simulink library "lib_env"  (Simulink 7.7)
settings: Solver=ode45  StartTime=0.0  StopTime=10.0  RelTol=1e-3
undefined symbols (not defined in the file): ADSW, area, arm, CD, CGP, CR, Earth, earth_radius, ele, GE, GGSW, GPperturbationSW, I, J2, jd, pSR, q_ini, rem_mag, rem_magSW, SGP, SRPSW, TOLERANCE, UT1_UTC, w_ini, wE, WGS84
libraries: lib_util x20, aerolibutil x13, lib_env x10, lib_orbittrance x9, aerolibtransform2 x6, lib_astrodynamics x5, aerolibatmos2 x1, vrlib x1, aerolibgravity2 x1
(part 1 of 2)
settings Model: Creator=kkamiya  LastModifiedBy=yamaurashusaku

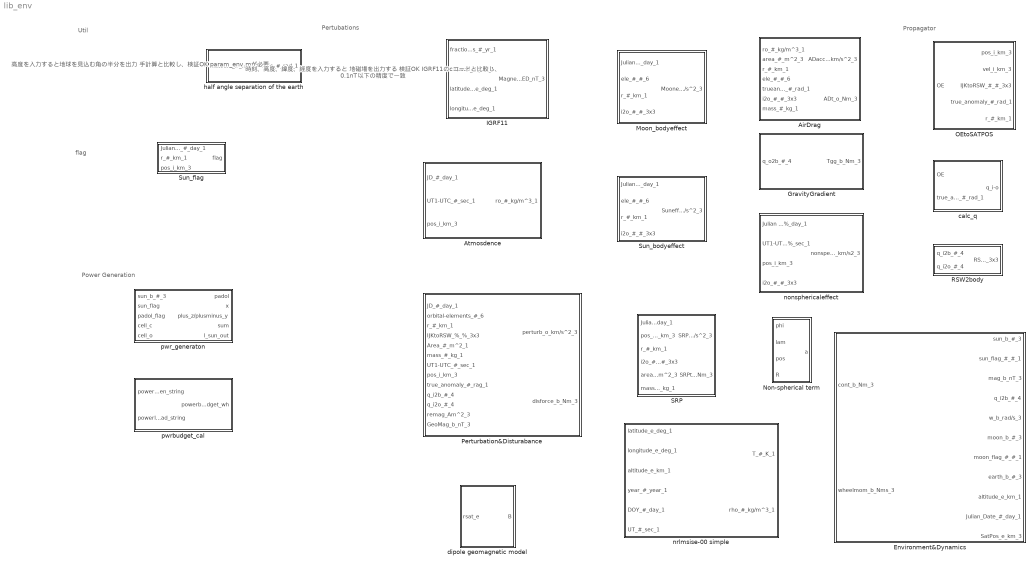
== system lib_env ==
  note: 高度を入力すると地球を見込む角の半分を出力
      | 手計算と比較し、検証OK
      | param_env.mが必要
  note: 時刻、高度、緯度、経度を入力すると
      | 地磁場を出力する
      | 検証OK
      | IGRF11のcコードと比較し、
      | 0.1nT以下の精度で一致
  note: Pertubations
  note: Util
  note: Propagator
  note: flag
  note: Power Generation
  AirDrag : Subsystem
  Atmosdence : Subsystem
  Environment&Dynamics : Subsystem
  GravityGradient : Subsystem
  IGRF11 : Subsystem
  Moon_bodyeffect : Subsystem
  Non-spherical term : Stateflow chart  TreatAsAtomicUnit=on
  OEtoSATPOS : Subsystem
  Perturbation&Disturabance : Subsystem
  RSW2body : Subsystem
  SRP : Subsystem
  Sun_bodyeffect : Subsystem
  Sun_flag : Subsystem
  calc_q : Subsystem
  dipole geomagnetic model : Stateflow chart  TreatAsAtomicUnit=on
  half angle separation of the earth : Subsystem
  nonsphericaleffect : Subsystem
  nrlmsise-00 simple : Subsystem
  pwr_generaton : Subsystem
  pwrbudget_cal : Subsystem

== system lib_env/AirDrag ==
  note: CD=2.2; arm=0.05cm
  ro_#_kg/m^3_1 : Inport
  area_#_m^2_3 : Inport  Port=2
  r_#_km_1 : Inport  Port=3
  ele_#_#_6 : Inport  Port=4
  trueanomaly_#_rad_1 : Inport  Port=5
  i2o_#_#_3x3 : Inport  Port=6
  mass_#_kg_1 : Inport  Port=7
  calc_AD : Stateflow chart  TreatAsAtomicUnit=on
  ADacc_o_km/s^2_3 : Outport
  ADt_o_Nm_3 : Outport  Port=2
  wires:
  calc_AD/1(AD_acc) -> ADacc_o_km/s^2_3/1
  calc_AD/2(AD_t) -> ADt_o_Nm_3/1
  ro_#_kg/m^3_1/1 -> calc_AD/1(ro)
  area_#_m^2_3/1 -> calc_AD/2(area)
  r_#_km_1/1 -> calc_AD/3(r)
  ele_#_#_6/1 -> calc_AD/4(ele)
  trueanomaly_#_rad_1/1 -> calc_AD/5(th)
  i2o_#_#_3x3/1 -> calc_AD/6(R)
  mass_#_kg_1/1 -> calc_AD/7(mass)

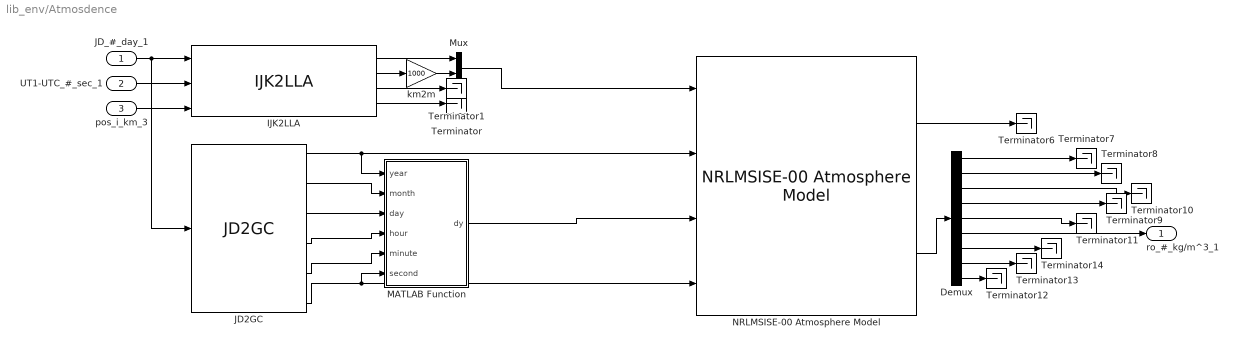
== system lib_env/Atmosdence ==
  JD_#_day_1 : Inport
  UT1-UTC_#_sec_1 : Inport  Port=2
  pos_i_km_3 : Inport  Port=3
  Demux : Demux  Outputs=9
  IJK2LLA : lib_orbittrance/IJK2LLA
  JD2GC : lib_util/JD2GC
  MATLAB Function : Stateflow chart  TreatAsAtomicUnit=on
  Mux : Mux  Inputs=2
  NRLMSISE-00 Atmosphere Model : aerolibatmos2/NRLMSISE-00 Atmosphere Model  units=Metric (MKS)  lst_input=off  flux_ap_input=off  flags_input=Internal  flags=ones(1,23)  oxygen_in=off  action=Warning
  Terminator{,1,6..14} (11 alike) : Terminator
  km2m : Gain  Gain=1000
  ro_#_kg/m^3_1 : Outport
  wires:
  IJK2LLA/1 -> Mux/1
  IJK2LLA/2 -> km2m/1
  km2m/1 -> Mux/2
  Mux/1 -> NRLMSISE-00 Atmosphere Model/1
  JD2GC/1 -> NRLMSISE-00 Atmosphere Model/2, MATLAB Function/1(year)
  JD2GC/6 -> NRLMSISE-00 Atmosphere Model/4, MATLAB Function/6(second)
  IJK2LLA/4 -> Terminator/1
  IJK2LLA/3 -> Terminator1/1
  JD2GC/2 -> MATLAB Function/2(month)
  JD2GC/3 -> MATLAB Function/3(day)
  JD2GC/4 -> MATLAB Function/4(hour)
  JD2GC/5 -> MATLAB Function/5(minute)
  JD_#_day_1/1 -> IJK2LLA/1, JD2GC/1
  UT1-UTC_#_sec_1/1 -> IJK2LLA/2
  pos_i_km_3/1 -> IJK2LLA/3
  NRLMSISE-00 Atmosphere Model/1 -> Terminator6/1
  NRLMSISE-00 Atmosphere Model/2 -> Demux/1
  Demux/6 -> ro_#_kg/m^3_1/1
  Demux/1 -> Terminator7/1
  Demux/2 -> Terminator8/1
  Demux/4 -> Terminator9/1
  Demux/3 -> Terminator10/1
  Demux/5 -> Terminator11/1
  Demux/9 -> Terminator12/1
  Demux/8 -> Terminator13/1
  Demux/7 -> Terminator14/1
  MATLAB Function/1(dy) -> NRLMSISE-00 Atmosphere Model/3

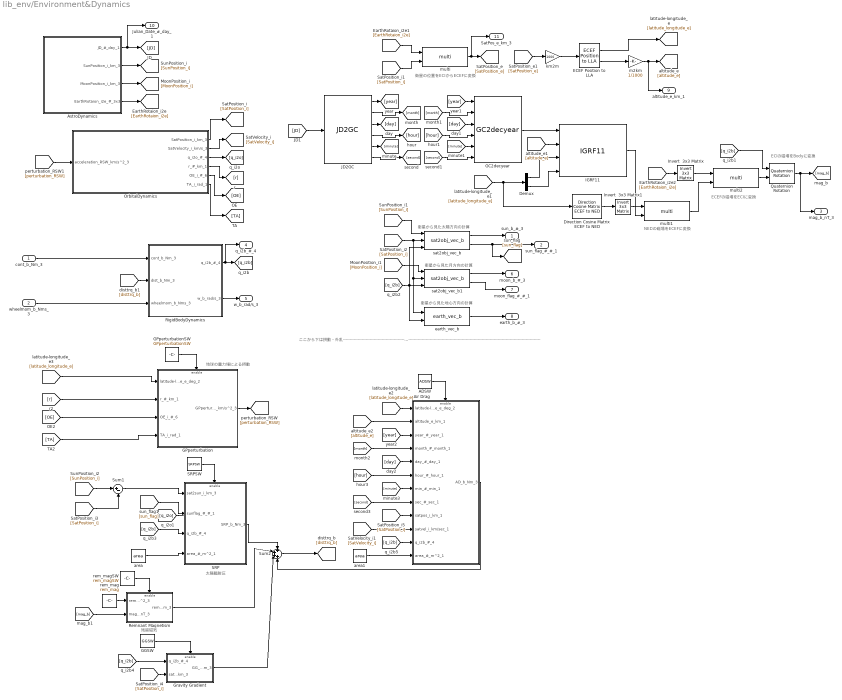
== system lib_env/Environment&Dynamics ==
  note: 残留磁気
  note: 太陽輻射圧
  note: 地球の重力場による摂動
  note: 衛星から見た地心方向の計算
  note: 衛星から見た月方向の計算
  note: 衛星から見た太陽方向の計算
  note: ECIの磁場をBodyに変換
  note: ECEFの磁場をECIに変換
  note: NEDの磁場をECEFに変換
  note: 衛星の位置をECIからECEFに変換
  note: ここから下は摂動・外乱-------------------------------------------------------------------------------------------------------------------------------------------------------------------------------------------------------------------------------------------------------------------------------------------------------------------------------------------------------
  cont_b_Nm_3 : Inport
  wheelmom_b_Nms_3 : Inport  Port=2
  ADSW : Constant  Value=ADSW
  Air Drag : Subsystem
  AstroDynamics : Subsystem
  Demux : Demux  Outputs=2
  Direction Cosine Matrix ECEF to NED : aerolibtransform2/Direction Cosine Matrix ECEF to NED  SystemSampleTime=-1
  ECEF Position to LLA : aerolibtransform2/ECEF Position to LLA  SystemSampleTime=-1  units=Metric (MKS)  ptype=Earth (WGS84)  F=1/298.257223563  R=6378137
  GC2decyear : lib_util/GC2decyear  SystemSampleTime=-1
  GGSW : Constant  Value=GGSW
  GPperturbation : Subsystem
  GPperturbationSW : Constant  Value=GPperturbationSW
  Gravity Gradient : Subsystem
  IGRF11 : lib_env/IGRF11  SystemSampleTime=-1
  Invert  3x3 Matrix : aerolibutil/Invert  3x3 Matrix  SystemSampleTime=-1
  Invert  3x3 Matrix1 : aerolibutil/Invert  3x3 Matrix  SystemSampleTime=-1
  JD2GC : lib_util/JD2GC  SystemSampleTime=-1
  OrbitalDynamics : Subsystem
  Quaternion Rotation : aerolibutil/Quaternion Rotation  SystemSampleTime=-1
  Remnant Magnetism : Subsystem
  RigidBodyDynamics : Subsystem
  SRP : Subsystem
  SRPSW : Constant  Value=SRPSW
  Sum1 : Sum  Inputs=|+-
  Sum2 : Sum  Inputs=++++
  area : Constant  Value=area
  area1 : Constant  Value=area
  earth_vec_b : lib_orbittrance/earth_vec_b  SystemSampleTime=-1
  km2m : Gain  Gain=1000
  m2km : Gain  Gain=1/1000
  multi : lib_util/multi  SystemSampleTime=-1
  multi1 : lib_util/multi  SystemSampleTime=-1
  multi2 : lib_util/multi  SystemSampleTime=-1
  rem_mag : Constant  Value=rem_mag
  rem_magSW : Constant  Value=rem_magSW
  sat2obj_vec_b : lib_orbittrance/sat2obj_vec_b  SystemSampleTime=-1
  sat2obj_vec_b1 : lib_orbittrance/sat2obj_vec_b  SystemSampleTime=-1
  sun_b_#_3 : Outport
  sun_flag_#_#_1 : Outport  Port=2
  mag_b_nT_3 : Outport  Port=3
  q_i2b_#_4 : Outport  Port=4
  w_b_rad/s_3 : Outport  Port=5
  moon_b_#_3 : Outport  Port=6
  moon_flag_#_#_1 : Outport  Port=7
  earth_b_#_3 : Outport  Port=8
  altitude_e_km_1 : Outport  Port=9
  Julian_Date_#_day_1 : Outport  Port=10
  SatPos_e_km_3 : Outport  Port=11
  wires:
  RigidBodyDynamics/2(w_b_rad/s_3) -> w_b_rad/s_3/1
  earth_vec_b/1 -> earth_b_#_3/1
  sat2obj_vec_b1/2 -> moon_flag_#_#_1/1
  sat2obj_vec_b1/1 -> moon_b_#_3/1
  sat2obj_vec_b/1 -> sun_b_#_3/1
  Air Drag/1(AD_b_Nm_3) -> Sum2/4
  ADSW/1 -> Air Drag/Enable
  [year] -> Air Drag/3(year_#_year_1)
  [q_i2b] -> Air Drag/11(q_i2b_#_4)
  area1/1 -> Air Drag/12(area_#_m^2_1)
  [SatVelocity_i] -> Air Drag/10(satvel_i_km/sec_1)
  [SatPosition_i] -> Air Drag/9(satpos_i_km_1)
  [second] -> Air Drag/8(sec_#_sec_1)
  [minute] -> Air Drag/7(min_#_min_1)
  [hour] -> Air Drag/6(hour_#_hour_1)
  [day] -> Air Drag/5(day_#_day_1)
  [month] -> Air Drag/4(month_#_month_1)
  [altitude_e] -> Air Drag/2(altitude_e_km_1)
  [latitude_longitude_e] -> Air Drag/1(latitude-longitude_e_deg_2)
  GGSW/1 -> Gravity Gradient/Enable
  [SatPosition_i] -> Gravity Gradient/2(satpos_i_km_3)
  [q_i2b] -> Gravity Gradient/1(q_i2b_#_4)
  SRP/1(SRP_b_Nm_3) -> Sum2/1
  [disttrq_b] -> RigidBodyDynamics/2(dist_b_Nm_3)
  Sum2/1 -> [disttrq_b]
  rem_magSW/1 -> Remnant Magnetism/Enable
  [mag_b] -> Remnant Magnetism/2(mag_b_nT_3)
  rem_mag/1 -> Remnant Magnetism/1(remmag_b_Am^2_3)
  SRPSW/1 -> SRP/Enable
  [SunPosition_i] -> Sum1/1
  [SatPosition_i] -> Sum1/2
  [q_i2b] -> SRP/3(q_i2b_#_4)
  [q_i2o] -> ?
  area/1 -> SRP/4(area_#_m^2_1)
  [sun_flag] -> SRP/2(sunflag_#_#_1)
  Sum1/1 -> SRP/1(sat2sun_i_km_3)
  sat2obj_vec_b/2 -> sun_flag_#_#_1/1, [sun_flag]
  [second] -> GC2decyear/6
  [minute] -> GC2decyear/5
  [hour] -> GC2decyear/4
  [day] -> GC2decyear/3
  [month] -> GC2decyear/2
  [year] -> GC2decyear/1
  JD2GC/6 -> [second]
  JD2GC/5 -> [minute]
  JD2GC/4 -> [hour]
  JD2GC/3 -> [day]
  JD2GC/2 -> [month]
  JD2GC/1 -> [year]
  GPperturbationSW/1 -> GPperturbation/Enable
  [TA] -> GPperturbation/4(TA_i_rad_1)
  [OE] -> GPperturbation/3(OE_i_#_6)
  [r] -> GPperturbation/2(r_#_km_1)
  [latitude_longitude_e] -> GPperturbation/1(latitude-longitude_e_deg_2)
  OrbitalDynamics/4(r_#_km_1) -> [r]
  OrbitalDynamics/6(TA_i_rad_1) -> [TA]
  OrbitalDynamics/5(OE_i_#_6) -> [OE]
  OrbitalDynamics/3(q_i2o_#_4) -> [q_i2o]
  [SunPosition_i] -> sat2obj_vec_b/1
  [MoonPosition_i] -> sat2obj_vec_b1/1
  [q_i2b] -> sat2obj_vec_b1/3, sat2obj_vec_b/3, earth_vec_b/2
  [SatPosition_i] -> sat2obj_vec_b/2, sat2obj_vec_b1/2, earth_vec_b/1
  Quaternion Rotation/1 -> mag_b_nT_3/1, [mag_b]
  [q_i2b] -> Quaternion Rotation/1
  RigidBodyDynamics/1(q_i2b_#_4) -> q_i2b_#_4/1, [q_i2b]
  multi2/1 -> Quaternion Rotation/2
  multi1/1 -> multi2/2
  Invert  3x3 Matrix/1 -> multi2/1
  [EarthRotaion_i2e] -> Invert  3x3 Matrix/1
  IGRF11/1 -> multi1/2
  Invert  3x3 Matrix1/1 -> multi1/1
  Direction Cosine Matrix ECEF to NED/1 -> Invert  3x3 Matrix1/1
  Demux/2 -> IGRF11/4
  Demux/1 -> IGRF11/3
  [altitude_e] -> IGRF11/2
  [latitude_longitude_e] -> Direction Cosine Matrix ECEF to NED/1, Demux/1
  [JD] -> JD2GC/1
  AstroDynamics/1(JD_#_day_1) -> Julian_Date_#_day_1/1, [JD]
  GC2decyear/1 -> IGRF11/1
  ECEF Position to LLA/1 -> [latitude_longitude_e]
  m2km/1 -> altitude_e_km_1/1, [altitude_e]
  ECEF Position to LLA/2 -> m2km/1
  km2m/1 -> ECEF Position to LLA/1
  [SatPosition_e] -> km2m/1
  multi/1 -> SatPos_e_km_3/1, [SatPosition_e]
  [SatPosition_i] -> multi/2
  [EarthRotaion_i2e] -> multi/1
  OrbitalDynamics/2(SatVelocity_i_km/s_3) -> [SatVelocity_i]
  OrbitalDynamics/1(SatPosition_i_km_3) -> [SatPosition_i]
  AstroDynamics/4(EarthRotaion_i2e_#_3x3) -> [EarthRotaion_i2e]
  AstroDynamics/3(MoonPosition_i_km_3) -> [MoonPosition_i]
  AstroDynamics/2(SunPosition_i_km_3) -> [SunPosition_i]
  wheelmom_b_Nms_3/1 -> RigidBodyDynamics/3(wheelmom_b_Nms_3)
  cont_b_Nm_3/1 -> RigidBodyDynamics/1(cont_b_Nm_3)
  Remnant Magnetism/1(remmag_b_Nm_3) -> Sum2/2
  Gravity Gradient/1(GG_b_Nm_3) -> Sum2/3
  GPperturbation/1(GPperturbation_RSW_km/s^2_3) -> [perturbation_RSW]
  [perturbation_RSW] -> OrbitalDynamics/1(acceleration_RSW_km/s^2_3)

== system lib_env/GravityGradient ==
  q_o2b_#_4 : Inport
  gravity_gradient : Stateflow chart  TreatAsAtomicUnit=on
  iInertiamatrix_#_kgm^2_3x3 : Constant  Value=I
  radius_vec : Stateflow chart  TreatAsAtomicUnit=on
  Tgg_b_Nm_3 : Outport
  wires:
  gravity_gradient/1(Tgg) -> Tgg_b_Nm_3/1
  radius_vec/1(ra_vec) -> gravity_gradient/1(ra)
  q_o2b_#_4/1 -> radius_vec/1(q)
  iInertiamatrix_#_kgm^2_3x3/1 -> gravity_gradient/2(I)

== system lib_env/IGRF11 ==
  fractional years_#_yr_1 : Inport
  altitude_#_km_1 : Inport  Port=2
  latitude_e_deg_1 : Inport  Port=3
  longitude_e_deg_1 : Inport  Port=4
  IGRF11 : Stateflow chart  TreatAsAtomicUnit=on
  Magnetic field_NED_nT_3 : Outport
  wires:
  fractional years_#_yr_1/1 -> IGRF11/1(fyears)
  altitude_#_km_1/1 -> IGRF11/2(alt)
  latitude_e_deg_1/1 -> IGRF11/3(nlat)
  longitude_e_deg_1/1 -> IGRF11/4(elong)
  IGRF11/1(B) -> Magnetic field_NED_nT_3/1

== system lib_env/Moon_bodyeffect ==
  JulianDate_#_day_1 : Inport
  ele_#_#_6 : Inport  Port=2
  r_#_km_1 : Inport  Port=3
  i2o_#_#_3x3 : Inport  Port=4
  moon position vector : lib_astrodynamics/moon position vector
  moonbodyeffect : Stateflow chart  TreatAsAtomicUnit=on
  Mooneff_o_km/s^2_3 : Outport
  wires:
  JulianDate_#_day_1/1 -> moon position vector/1
  r_#_km_1/1 -> moonbodyeffect/5(r)
  ele_#_#_6/1 -> moonbodyeffect/4(ele)
  i2o_#_#_3x3/1 -> moonbodyeffect/6(R)
  moonbodyeffect/1(F) -> Mooneff_o_km/s^2_3/1
  moon position vector/1 -> moonbodyeffect/1(lon)
  moon position vector/2 -> moonbodyeffect/2(lat)
  moon position vector/3 -> moonbodyeffect/3(rp)

== system lib_env/OEtoSATPOS ==
  OE : Inport
  calc_TA_R : Stateflow chart  TreatAsAtomicUnit=on
  sat_IJK : Stateflow chart  TreatAsAtomicUnit=on
  pos_i_km_3 : Outport
  vel_i_km_3 : Outport  Port=2
  IJKtoRSW_#_#_3x3 : Outport  Port=3
  true_anomaly_#_rad_1 : Outport  Port=4
  r_#_km_1 : Outport  Port=5
  wires:
  OE/1 -> calc_TA_R/1(OE)
  calc_TA_R/1(ele) -> sat_IJK/1(ele)
  calc_TA_R/2(th) -> sat_IJK/2(th), true_anomaly_#_rad_1/1
  calc_TA_R/3(r) -> sat_IJK/3(r), r_#_km_1/1
  calc_TA_R/4(R) -> sat_IJK/4(R), IJKtoRSW_#_#_3x3/1
  sat_IJK/1(pos) -> pos_i_km_3/1
  sat_IJK/2(v) -> vel_i_km_3/1

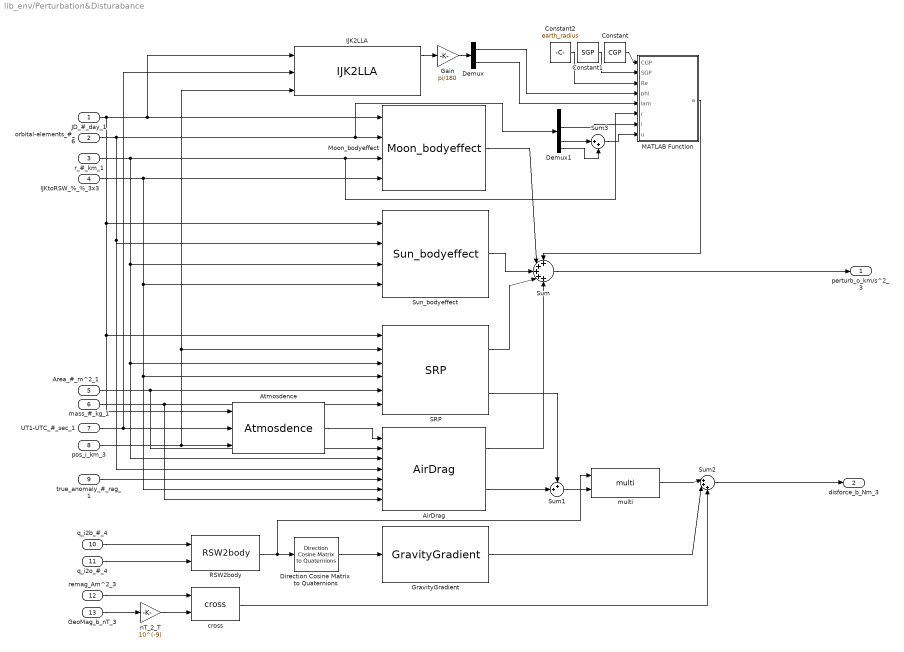
== system lib_env/Perturbation&Disturabance ==
  JD_#_day_1 : Inport
  orbital-elements_#_6 : Inport  Port=2
  r_#_km_1 : Inport  Port=3
  IJKtoRSW_%_%_3x3 : Inport  Port=4
  Area_#_m^2_1 : Inport  Port=5
  mass_#_kg_1 : Inport  Port=6
  UT1-UTC_#_sec_1 : Inport  Port=7
  pos_i_km_3 : Inport  Port=8
  true_anomaly_#_rag_1 : Inport  Port=9
  q_i2b_#_4 : Inport  Port=10
  q_i2o_#_4 : Inport  Port=11
  remag_Am^2_3 : Inport  Port=12
  GeoMag_b_nT_3 : Inport  Port=13
  AirDrag : lib_env/AirDrag
  Atmosdence : lib_env/Atmosdence
  Constant : Constant  Value=CGP
  Constant1 : Constant  Value=SGP
  Constant2 : Constant  Value=earth_radius
  Demux : Demux  Outputs=2
  Demux1 : Demux  Outputs=6
  Direction Cosine Matrix  to Quaternions : aerolibtransform2/Direction Cosine Matrix  to Quaternions
  Gain : Gain  Gain=pi/180
  GravityGradient : lib_env/GravityGradient
  IJK2LLA : lib_orbittrance/IJK2LLA
  MATLAB Function : Stateflow chart  TreatAsAtomicUnit=on
  Moon_bodyeffect : lib_env/Moon_bodyeffect
  RSW2body : lib_env/RSW2body
  SRP : lib_env/SRP
  Sum : Sum  Inputs=+++++
  Sum1 : Sum  Inputs=++|
  Sum2 : Sum  Inputs=|+++
  Sum3 : Sum  Inputs=|++
  Sun_bodyeffect : lib_env/Sun_bodyeffect
  cross : lib_util/cross
  multi : lib_util/multi
  nT_2_T : Gain  Gain=10^(-9)
  perturb_o_km/s^2_3 : Outport
  disforce_b_Nm_3 : Outport  Port=2
  wires:
  JD_#_day_1/1 -> Sun_bodyeffect/1, SRP/1, Atmosdence/1, Moon_bodyeffect/1, IJK2LLA/1
  orbital-elements_#_6/1 -> Sun_bodyeffect/2, AirDrag/4, Moon_bodyeffect/2, Demux1/1
  r_#_km_1/1 -> Sun_bodyeffect/3, SRP/3, AirDrag/3, Moon_bodyeffect/3, MATLAB Function/6(r)
  IJKtoRSW_%_%_3x3/1 -> Sun_bodyeffect/4, SRP/4, AirDrag/6, Moon_bodyeffect/4
  Area_#_m^2_1/1 -> SRP/5, AirDrag/2
  mass_#_kg_1/1 -> SRP/6, AirDrag/7
  true_anomaly_#_rag_1/1 -> AirDrag/5
  Sum/1 -> perturb_o_km/s^2_3/1
  SRP/2 -> Sum1/1
  AirDrag/2 -> Sum1/2
  Atmosdence/1 -> AirDrag/1
  UT1-UTC_#_sec_1/1 -> IJK2LLA/2, Atmosdence/2
  pos_i_km_3/1 -> Atmosdence/3, IJK2LLA/3, SRP/2
  q_i2b_#_4/1 -> RSW2body/1
  q_i2o_#_4/1 -> RSW2body/2
  RSW2body/1 -> Direction Cosine Matrix  to Quaternions/1, multi/1
  Direction Cosine Matrix  to Quaternions/1 -> GravityGradient/1
  GravityGradient/1 -> Sum2/2
  Sum1/1 -> multi/2
  multi/1 -> Sum2/1
  AirDrag/1 -> Sum/5
  SRP/1 -> Sum/4
  Sun_bodyeffect/1 -> Sum/3
  Moon_bodyeffect/1 -> Sum/2
  Sum2/1 -> disforce_b_Nm_3/1
  IJK2LLA/1 -> Gain/1
  Gain/1 -> Demux/1
  GeoMag_b_nT_3/1 -> nT_2_T/1
  nT_2_T/1 -> cross/2
  remag_Am^2_3/1 -> cross/1
  cross/1 -> Sum2/3
  Constant/1 -> MATLAB Function/1(CGP)
  Constant1/1 -> MATLAB Function/2(SGP)
  Constant2/1 -> MATLAB Function/3(Re)
  Demux/1 -> MATLAB Function/4(phi)
  Demux/2 -> MATLAB Function/5(lam)
  MATLAB Function/1(a) -> Sum/1
  Demux1/3 -> MATLAB Function/7(i)
  Demux1/5 -> Sum3/1
  Demux1/6 -> Sum3/2
  Sum3/1 -> MATLAB Function/8(u)

== system lib_env/RSW2body ==
  q_i2b_#_4 : Inport
  q_i2o_#_4 : Inport  Port=2
  Invert  3x3 Matrix : aerolibutil/Invert  3x3 Matrix
  Quaternions to  Direction Cosine Matrix : aerolibtransform2/Quaternions to  Direction Cosine Matrix
  Quaternions to  Direction Cosine Matrix1 : aerolibtransform2/Quaternions to  Direction Cosine Matrix
  multi : lib_util/multi
  RSW2b_#_#_3x3 : Outport
  wires:
  q_i2b_#_4/1 -> Quaternions to  Direction Cosine Matrix/1
  q_i2o_#_4/1 -> Quaternions to  Direction Cosine Matrix1/1
  Quaternions to  Direction Cosine Matrix1/1 -> Invert  3x3 Matrix/1
  Invert  3x3 Matrix/1 -> multi/2
  Quaternions to  Direction Cosine Matrix/1 -> multi/1
  multi/1 -> RSW2b_#_#_3x3/1

== system lib_env/SRP ==
  note: Arm=0.05cm
  JulianDate_#_day_1 : Inport
  pos_#_km_3 : Inport  Port=2
  r_#_km_1 : Inport  Port=3
  i2o_#_#_3x3 : Inport  Port=4
  area_#_m^2_3 : Inport  Port=5
  mass_#_kg_1 : Inport  Port=6
  srp : Stateflow chart  TreatAsAtomicUnit=on
  SRP_o_km/s^2_3 : Outport
  SRPt_o_Nm_3 : Outport  Port=2
  wires:
  r_#_km_1/1 -> srp/3(r)
  pos_#_km_3/1 -> srp/2(pos)
  i2o_#_#_3x3/1 -> srp/4(R)
  srp/1(SRP_acc) -> SRP_o_km/s^2_3/1
  JulianDate_#_day_1/1 -> srp/1(jd)
  area_#_m^2_3/1 -> srp/5(area)
  mass_#_kg_1/1 -> srp/6(mass)
  srp/2(SRP_t) -> SRPt_o_Nm_3/1

== system lib_env/Sun_bodyeffect ==
  JulianDate_#_day_1 : Inport
  ele_#_#_6 : Inport  Port=2
  r_#_km_1 : Inport  Port=3
  i2o_#_#_3x3 : Inport  Port=4
  Sun : lib_astrodynamics/sun position vector/Sun
  sun_b_e : Stateflow chart  TreatAsAtomicUnit=on
  Suneff_o_km/s^2_3 : Outport
  wires:
  Sun/1 -> sun_b_e/1(lon)
  Sun/2 -> sun_b_e/2(lat)
  Sun/3 -> sun_b_e/3(rp)
  r_#_km_1/1 -> sun_b_e/5(r)
  ele_#_#_6/1 -> sun_b_e/4(ele)
  i2o_#_#_3x3/1 -> sun_b_e/6(R)
  sun_b_e/1(F) -> Suneff_o_km/s^2_3/1
  JulianDate_#_day_1/1 -> Sun/1

== system lib_env/Sun_flag ==
  JulianDate_#_day_1 : Inport
  r_#_km_1 : Inport  Port=2
  pos_i_km_3 : Inport  Port=3
  srp : Stateflow chart  TreatAsAtomicUnit=on
  flag : Outport
  wires:
  pos_i_km_3/1 -> srp/2(pos)
  r_#_km_1/1 -> srp/3(r)
  srp/1(flag) -> flag/1
  JulianDate_#_day_1/1 -> srp/1(jd)

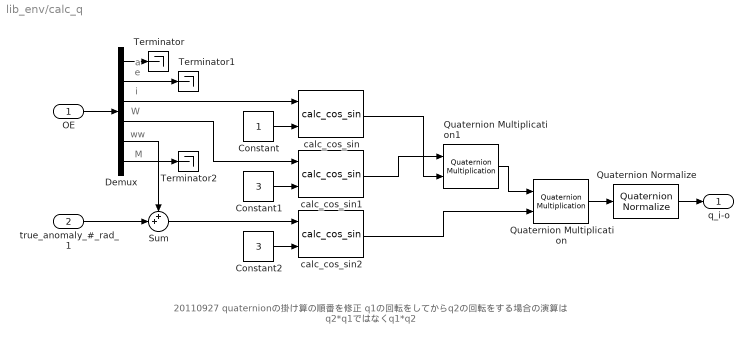
== system lib_env/calc_q ==
  note: M
  note: ww
  note: W
  note: i
  note: e
  note: a
  note: 20110927 quaternionの掛け算の順番を修正
      | q1の回転をしてからq2の回転をする場合の演算は
      | q2*q1ではなくq1*q2
  OE : Inport
  true_anomaly_#_rad_1 : Inport  Port=2
  Constant : Constant
  Constant1 : Constant  Value=3
  Constant2 : Constant  Value=3
  Demux : Demux  Outputs=6
  Quaternion Multiplication : aerolibutil/Quaternion Multiplication
  Quaternion Multiplication1 : aerolibutil/Quaternion Multiplication
  Quaternion Normalize : aerolibutil/Quaternion Normalize
  Sum : Sum  Inputs=++|
  Terminator : Terminator
  Terminator1 : Terminator
  Terminator2 : Terminator
  calc_cos_sin : lib_util/calc_cos_sin
  calc_cos_sin1 : lib_util/calc_cos_sin
  calc_cos_sin2 : lib_util/calc_cos_sin
  q_i-o : Outport
  wires:
  OE/1 -> Demux/1
  Quaternion Normalize/1 -> q_i-o/1
  true_anomaly_#_rad_1/1 -> Sum/2
  Demux/5 -> Sum/1
  Sum/1 -> calc_cos_sin2/1
  Demux/3 -> calc_cos_sin/1
  Demux/4 -> calc_cos_sin1/1
  Demux/1 -> Terminator/1
  Demux/2 -> Terminator1/1
  Demux/6 -> Terminator2/1
  Quaternion Multiplication/1 -> Quaternion Normalize/1
  Constant/1 -> calc_cos_sin/2
  Constant1/1 -> calc_cos_sin1/2
  Constant2/1 -> calc_cos_sin2/2
  calc_cos_sin1/1 -> Quaternion Multiplication1/1
  calc_cos_sin/1 -> Quaternion Multiplication1/2
  Quaternion Multiplication1/1 -> Quaternion Multiplication/1
  calc_cos_sin2/1 -> Quaternion Multiplication/2

== system lib_env/half angle separation of the earth ==
  altitude_#_km_1 : Inport
  MATLAB Function : Stateflow chart  TreatAsAtomicUnit=on
  earth radius_#_km_1 : Constant  Value=earth_radius
  angle_#_rad_1 : Outport
  wires:
  earth radius_#_km_1/1 -> MATLAB Function/2(R)
  altitude_#_km_1/1 -> MATLAB Function/1(h)
  MATLAB Function/1(ang) -> angle_#_rad_1/1

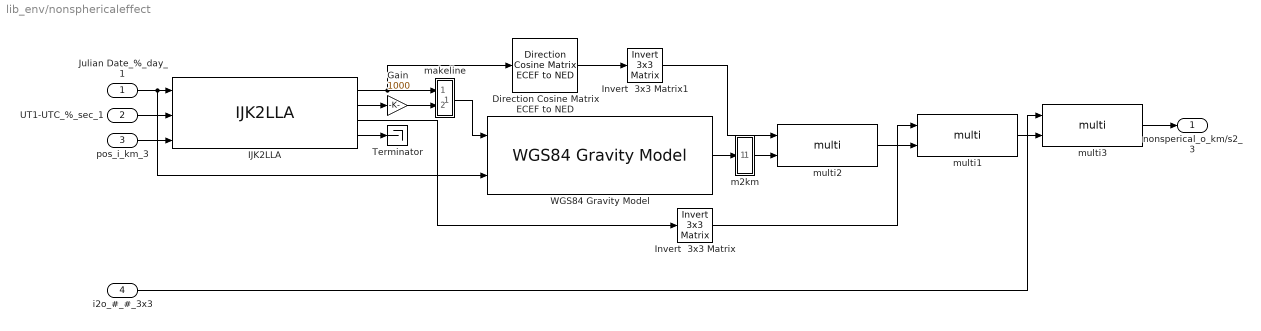
== system lib_env/nonsphericaleffect ==
  Julian Date_%_day_1 : Inport
  UT1-UTC_%_sec_1 : Inport  Port=2
  pos_i_km_3 : Inport  Port=3
  i2o_#_#_3x3 : Inport  Port=4
  Direction Cosine Matrix ECEF to NED : aerolibtransform2/Direction Cosine Matrix ECEF to NED
  Gain : Gain  Gain=1000
  IJK2LLA : lib_orbittrance/IJK2LLA
  Invert  3x3 Matrix : aerolibutil/Invert  3x3 Matrix
  Invert  3x3 Matrix1 : aerolibutil/Invert  3x3 Matrix
  Terminator : Terminator
  "WGS84 Gravity Model " : aerolibgravity2/WGS84 Gravity Model   model=WGS84 Exact  units=Metric (MKS)  no_atmos=on  precessing=on  jd_loc=on  month=October  day=10  year=2004  no_centrifugal=on  action=Warning
  m2km : Stateflow chart  TreatAsAtomicUnit=on
  makeline : Stateflow chart  TreatAsAtomicUnit=on
  multi1 : lib_util/multi
  multi2 : lib_util/multi
  multi3 : lib_util/multi
  nonsperical_o_km/s2_3 : Outport
  wires:
  IJK2LLA/1 -> Direction Cosine Matrix ECEF to NED/1, makeline/1(u)
  makeline/1(y) -> "WGS84 Gravity Model "/1
  Direction Cosine Matrix ECEF to NED/1 -> Invert  3x3 Matrix1/1
  "WGS84 Gravity Model "/1 -> m2km/1(u)
  IJK2LLA/3 -> Invert  3x3 Matrix/1
  Gain/1 -> makeline/2(v)
  IJK2LLA/2 -> Gain/1
  m2km/1(y) -> multi2/2
  Invert  3x3 Matrix/1 -> multi1/1
  multi2/1 -> multi1/2
  Invert  3x3 Matrix1/1 -> multi2/1
  Julian Date_%_day_1/1 -> IJK2LLA/1, "WGS84 Gravity Model "/2
  UT1-UTC_%_sec_1/1 -> IJK2LLA/2
  pos_i_km_3/1 -> IJK2LLA/3
  IJK2LLA/4 -> Terminator/1
  i2o_#_#_3x3/1 -> multi3/1
  multi1/1 -> multi3/2
  multi3/1 -> nonsperical_o_km/s2_3/1

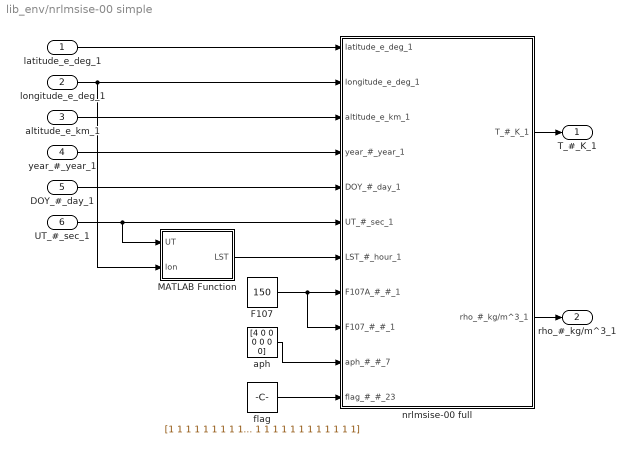
== system lib_env/nrlmsise-00 simple ==
  latitude_e_deg_1 : Inport
  longitude_e_deg_1 : Inport  Port=2
  altitude_e_km_1 : Inport  Port=3
  year_#_year_1 : Inport  Port=4
  DOY_#_day_1 : Inport  Port=5
  UT_#_sec_1 : Inport  Port=6
  F107 : Constant  Value=150
  MATLAB Function : Stateflow chart  TreatAsAtomicUnit=on
  aph : Constant  Value=[4 0 0 0 0 0 0]
  flag : Constant  Value=[1 1 1 1 1 1 1 1 1 1 1 1 1 1 1 1 1 1 1 1 1 1 1]
  nrlmsise-00 full : Subsystem
  T_#_K_1 : Outport
  rho_#_kg/m^3_1 : Outport  Port=2
  wires:
  longitude_e_deg_1/1 -> MATLAB Function/2(lon), nrlmsise-00 full/2(longitude_e_deg_1)
  UT_#_sec_1/1 -> MATLAB Function/1(UT), nrlmsise-00 full/6(UT_#_sec_1)
  flag/1 -> nrlmsise-00 full/11(flag_#_#_23)
  aph/1 -> nrlmsise-00 full/10(aph_#_#_7)
  F107/1 -> nrlmsise-00 full/8(F107A_#_#_1), nrlmsise-00 full/9(F107_#_#_1)
  MATLAB Function/1(LST) -> nrlmsise-00 full/7(LST_#_hour_1)
  latitude_e_deg_1/1 -> nrlmsise-00 full/1(latitude_e_deg_1)
  altitude_e_km_1/1 -> nrlmsise-00 full/3(altitude_e_km_1)
  nrlmsise-00 full/1(T_#_K_1) -> T_#_K_1/1
  year_#_year_1/1 -> nrlmsise-00 full/4(year_#_year_1)
  DOY_#_day_1/1 -> nrlmsise-00 full/5(DOY_#_day_1)
  nrlmsise-00 full/2(rho_#_kg/m^3_1) -> rho_#_kg/m^3_1/1

== system lib_env/pwr_generaton ==
  sun_b_#_3 : Inport
  sun_flag : Inport  Port=2
  padol_flag : Inport  Port=3
  cell_c : Inport  Port=4
  cell_o : Inport  Port=5
  Add : Sum  Inputs=+++
  solargeneration : Stateflow chart  TreatAsAtomicUnit=on
  padol : Outport
  x : Outport  Port=2
  plus_z/plusminus_y : Outport  Port=3
  sum : Outport  Port=4
  l_sun_out : Outport  Port=5
  wires:
  sun_flag/1 -> solargeneration/2(sun_flag)
  Add/1 -> sum/1
  sun_b_#_3/1 -> solargeneration/1(sun)
  solargeneration/1(padol) -> padol/1, Add/1
  solargeneration/2(x_p) -> x/1, Add/2
  solargeneration/3(z_y_p) -> plus_z/plusminus_y/1, Add/3
  solargeneration/4(l_sun_out) -> l_sun_out/1
  padol_flag/1 -> solargeneration/3(padol_flag)
  cell_c/1 -> solargeneration/4(cell_c)
  cell_o/1 -> solargeneration/5(cell_o)

== system lib_env/pwrbudget_cal ==
  powergen_string : Inport
  powerload_string : Inport  Port=2
  Efficiency : Stateflow chart  TreatAsAtomicUnit=on
  Integrator : Integrator
  Sum1 : Sum  Inputs=+-|
  pwrgenperstring : Gain  Gain=15.4
  pwrload : Stateflow chart  TreatAsAtomicUnit=on
  sec2hour : Gain  Gain=1/3600
  powerbudget_wh : Outport
  wires:
  powerload_string/1 -> pwrload/1(u)
  powergen_string/1 -> Sum1/1
  Sum1/1 -> Efficiency/1(u)
  Integrator/1 -> pwrgenperstring/1
  Efficiency/1(y) -> Integrator/1
  pwrgenperstring/1 -> sec2hour/1
  sec2hour/1 -> powerbudget_wh/1
  pwrload/1(p) -> Sum1/2

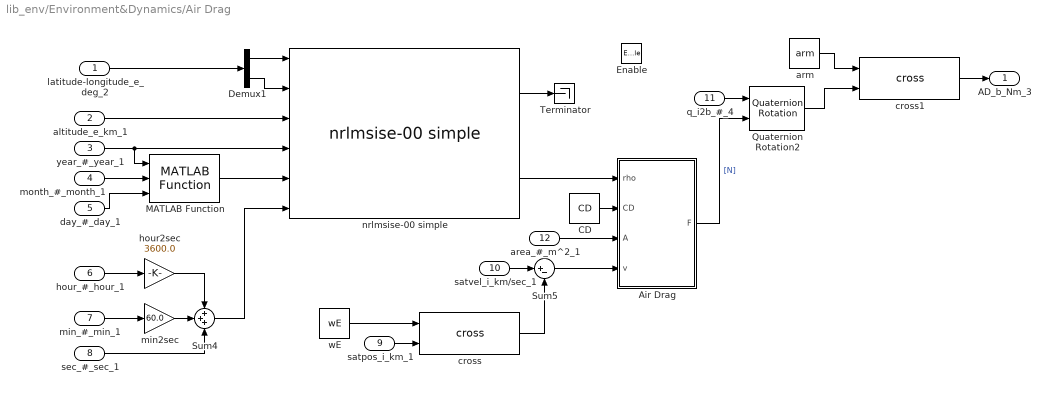
== system lib_env/Environment&Dynamics/Air Drag ==
  latitude-longitude_e_deg_2 : Inport
  altitude_e_km_1 : Inport  Port=2
  year_#_year_1 : Inport  Port=3
  month_#_month_1 : Inport  Port=4
  day_#_day_1 : Inport  Port=5
  hour_#_hour_1 : Inport  Port=6
  min_#_min_1 : Inport  Port=7
  sec_#_sec_1 : Inport  Port=8
  satpos_i_km_1 : Inport  Port=9
  satvel_i_km/sec_1 : Inport  Port=10
  q_i2b_#_4 : Inport  Port=11
  area_#_m^2_1 : Inport  Port=12
  Enable : EnablePort
  Air Drag : Stateflow chart  TreatAsAtomicUnit=on
  CD : Constant  Value=CD
  Demux1 : Demux  Outputs=2
  MATLAB Function : lib_util/MATLAB Function  SystemSampleTime=-1
  Quaternion Rotation2 : aerolibutil/Quaternion Rotation  SystemSampleTime=-1
  Sum4 : Sum  Inputs=+++
  Sum5 : Sum  Inputs=|+-
  Terminator : Terminator
  arm : Constant  Value=arm
  cross : lib_util/cross  SystemSampleTime=-1
  cross1 : lib_util/cross  SystemSampleTime=-1
  hour2sec : Gain  Gain=3600.0
  min2sec : Gain  Gain=60.0
  nrlmsise-00 simple : lib_env/nrlmsise-00 simple  SystemSampleTime=-1
  wE : Constant  Value=wE
  AD_b_Nm_3 : Outport
  wires:
  satpos_i_km_1/1 -> cross/2
  sec_#_sec_1/1 -> Sum4/3
  min_#_min_1/1 -> min2sec/1
  hour_#_hour_1/1 -> hour2sec/1
  satvel_i_km/sec_1/1 -> Sum5/1
  area_#_m^2_1/1 -> Air Drag/3(A)
  day_#_day_1/1 -> MATLAB Function/3
  month_#_month_1/1 -> MATLAB Function/2
  altitude_e_km_1/1 -> nrlmsise-00 simple/3
  q_i2b_#_4/1 -> Quaternion Rotation2/1
  cross1/1 -> AD_b_Nm_3/1
  arm/1 -> cross1/1
  latitude-longitude_e_deg_2/1 -> Demux1/1
  Quaternion Rotation2/1 -> cross1/2
  Air Drag/1(F) -> Quaternion Rotation2/2  "[N]"
  nrlmsise-00 simple/1 -> Terminator/1
  CD/1 -> Air Drag/2(CD)
  nrlmsise-00 simple/2 -> Air Drag/1(rho)
  Sum5/1 -> Air Drag/4(v)
  cross/1 -> Sum5/2
  wE/1 -> cross/1
  Sum4/1 -> nrlmsise-00 simple/6
  hour2sec/1 -> Sum4/1
  min2sec/1 -> Sum4/2
  year_#_year_1/1 -> MATLAB Function/1, nrlmsise-00 simple/4
  MATLAB Function/1 -> nrlmsise-00 simple/5
  Demux1/2 -> nrlmsise-00 simple/2
  Demux1/1 -> nrlmsise-00 simple/1

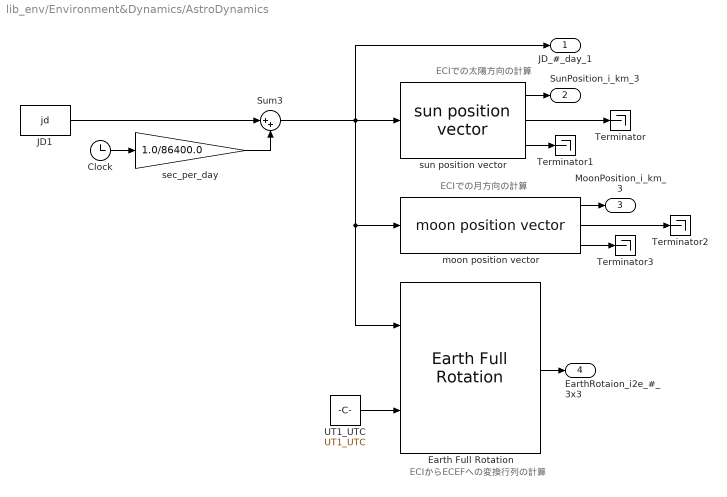
== system lib_env/Environment&Dynamics/AstroDynamics ==
  note: ECIからECEFへの変換行列の計算
  note: ECIでの月方向の計算
  note: ECIでの太陽方向の計算
  Clock : Clock
      settings: Decimation=10
  Earth Full Rotation : lib_astrodynamics/Earth Full Rotation  SystemSampleTime=-1
  JD1 : Constant  Value=jd
  Sum3 : Sum  Inputs=|++
  Terminator{,1..3} (4 alike) : Terminator
  UT1_UTC : Constant  Value=UT1_UTC  VectorParams1D=off
  moon position vector : lib_astrodynamics/moon position vector  SystemSampleTime=-1
  sec_per_day : Gain  Gain=1.0/86400.0
  sun position vector : lib_astrodynamics/sun position vector  SystemSampleTime=-1
  JD_#_day_1 : Outport
  SunPosition_i_km_3 : Outport  Port=2
  MoonPosition_i_km_3 : Outport  Port=3
  EarthRotaion_i2e_#_3x3 : Outport  Port=4
  wires:
  moon position vector/3 -> Terminator3/1
  moon position vector/2 -> Terminator2/1
  sun position vector/3 -> Terminator1/1
  sun position vector/2 -> Terminator/1
  Earth Full Rotation/1 -> EarthRotaion_i2e_#_3x3/1
  moon position vector/1 -> MoonPosition_i_km_3/1
  sun position vector/1 -> SunPosition_i_km_3/1
  UT1_UTC/1 -> Earth Full Rotation/2
  Sum3/1 -> JD_#_day_1/1, Earth Full Rotation/1, moon position vector/1, sun position vector/1
  Clock/1 -> sec_per_day/1
  sec_per_day/1 -> Sum3/2
  JD1/1 -> Sum3/1

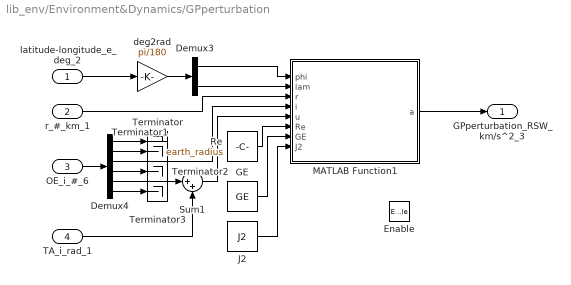
== system lib_env/Environment&Dynamics/GPperturbation ==
  latitude-longitude_e_deg_2 : Inport
  r_#_km_1 : Inport  Port=2
  OE_i_#_6 : Inport  Port=3
  TA_i_rad_1 : Inport  Port=4
  Enable : EnablePort
  Demux3 : Demux  Outputs=2
  Demux4 : Demux  Outputs=6
  GE : Constant  Value=GE
  J2 : Constant  Value=J2
  MATLAB Function1 : Stateflow chart  TreatAsAtomicUnit=on
  Re : Constant  Value=earth_radius
  Sum1 : Sum  Inputs=|++
  Terminator{,1..3} (4 alike) : Terminator
  deg2rad : Gain  Gain=pi/180
  GPperturbation_RSW_km/s^2_3 : Outport  InitialOutput=[0; 0; 0]
  wires:
  J2/1 -> MATLAB Function1/8(J2)
  TA_i_rad_1/1 -> Sum1/2
  OE_i_#_6/1 -> Demux4/1
  MATLAB Function1/1(a) -> GPperturbation_RSW_km/s^2_3/1
  r_#_km_1/1 -> MATLAB Function1/3(r)
  latitude-longitude_e_deg_2/1 -> deg2rad/1
  Demux4/6 -> Terminator3/1
  Demux4/4 -> Terminator2/1
  Demux4/2 -> Terminator1/1
  Demux4/1 -> Terminator/1
  GE/1 -> MATLAB Function1/7(GE)
  Re/1 -> MATLAB Function1/6(Re)
  Sum1/1 -> MATLAB Function1/5(u)
  Demux4/5 -> Sum1/1
  Demux4/3 -> MATLAB Function1/4(i)
  Demux3/2 -> MATLAB Function1/2(lam)
  Demux3/1 -> MATLAB Function1/1(phi)
  deg2rad/1 -> Demux3/1

== system lib_env/Environment&Dynamics/Gravity Gradient ==
  q_i2b_#_4 : Inport
  satpos_i_km_3 : Inport  Port=2
  Enable : EnablePort
  GE : Constant  Value=GE
  Inertiamatrix_#_kgm^2_3x3 : Constant  Value=I
  MATLAB Function : Stateflow chart  TreatAsAtomicUnit=on
  Quaternion Rotation1 : aerolibutil/Quaternion Rotation
  GG_b_Nm_3 : Outport  InitialOutput=[0; 0; 0]
  wires:
  MATLAB Function/1(T) -> GG_b_Nm_3/1
  satpos_i_km_3/1 -> Quaternion Rotation1/2
  q_i2b_#_4/1 -> Quaternion Rotation1/1
  Inertiamatrix_#_kgm^2_3x3/1 -> MATLAB Function/3(I)
  GE/1 -> MATLAB Function/2(GE)
  Quaternion Rotation1/1 -> MATLAB Function/1(R)

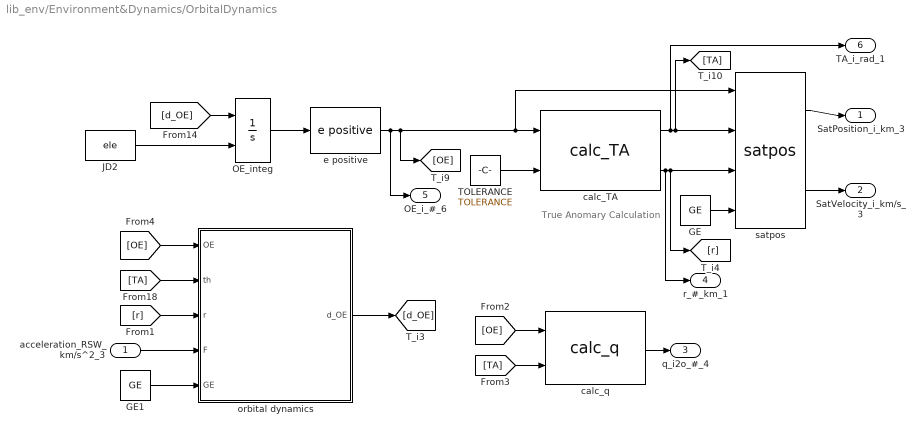
== system lib_env/Environment&Dynamics/OrbitalDynamics ==
  note: True Anomary
      | Calculation
  acceleration_RSW_km/s^2_3 : Inport
  GE : Constant  Value=GE
  GE1 : Constant  Value=GE
  JD2 : Constant  Value=ele  VectorParams1D=off
  OE_integ : Integrator  InitialConditionSource=external
  TOLERANCE : Constant  Value=TOLERANCE
  calc_TA : lib_orbittrance/calc_TA  SystemSampleTime=-1
  calc_q : lib_env/calc_q  SystemSampleTime=-1
  e positive : lib_orbittrance/e positive  SystemSampleTime=-1
  orbital dynamics : Stateflow chart  TreatAsAtomicUnit=on
  satpos : lib_orbittrance/satpos  SystemSampleTime=-1
  SatPosition_i_km_3 : Outport
  SatVelocity_i_km/s_3 : Outport  Port=2
  q_i2o_#_4 : Outport  Port=3
  r_#_km_1 : Outport  Port=4
  OE_i_#_6 : Outport  Port=5
  TA_i_rad_1 : Outport  Port=6
  wires:
  GE1/1 -> orbital dynamics/5(GE)
  acceleration_RSW_km/s^2_3/1 -> orbital dynamics/4(F)
  calc_q/1 -> q_i2o_#_4/1
  satpos/2 -> SatVelocity_i_km/s_3/1
  satpos/1 -> SatPosition_i_km_3/1
  [TA] -> calc_q/2
  GE/1 -> satpos/4
  calc_TA/2 -> r_#_km_1/1, satpos/3, [r]
  calc_TA/1 -> TA_i_rad_1/1, satpos/2, [TA]
  TOLERANCE/1 -> calc_TA/2
  [OE] -> calc_q/1
  orbital dynamics/1(d_OE) -> [d_OE]
  [r] -> orbital dynamics/3(r)
  [TA] -> orbital dynamics/2(th)
  OE_integ/1 -> e positive/1
  [OE] -> orbital dynamics/1(OE)
  [d_OE] -> OE_integ/1
  JD2/1 -> OE_integ/2
  e positive/1 -> satpos/1, calc_TA/1, [OE], OE_i_#_6/1

== system lib_env/Environment&Dynamics/Remnant Magnetism ==
  remmag_b_Am^2_3 : Inport
  mag_b_nT_3 : Inport  Port=2
  Enable : EnablePort
  cross : lib_util/cross  SystemSampleTime=-1
  nT2T : Gain  Gain=1.0e-9
  remmag_b_Nm_3 : Outport  InitialOutput=[0; 0; 0]
  wires:
  nT2T/1 -> cross/2
  mag_b_nT_3/1 -> nT2T/1
  cross/1 -> remmag_b_Nm_3/1
  remmag_b_Am^2_3/1 -> cross/1

== system lib_env/Environment&Dynamics/RigidBodyDynamics ==
  cont_b_Nm_3 : Inport
  dist_b_Nm_3 : Inport  Port=2
  wheelmom_b_Nms_3 : Inport  Port=3
  IC : InitialCondition  Value=[q_ini]
  IC1 : InitialCondition  Value=[w_ini]
  Integrator : Integrator  InitialCondition=q_ini
  Integrator1 : Integrator  InitialCondition=w_ini
  Quaternion Normalize : aerolibutil/Quaternion Normalize  SystemSampleTime=-1
  dynamics : Stateflow chart  TreatAsAtomicUnit=on
  iInertiamatrix_#_kgm^2_3x3 : Constant  Value=I
  q_i2b_#_4 : Outport
  w_b_rad/s_3 : Outport  Port=2
  wires:
  wheelmom_b_Nms_3/1 -> dynamics/5(hw)
  dist_b_Nm_3/1 -> dynamics/4(t_dist)
  iInertiamatrix_#_kgm^2_3x3/1 -> dynamics/6(I)
  Integrator1/1 -> IC1/1, w_b_rad/s_3/1
  dynamics/2(d_rate) -> Integrator1/1
  Integrator/1 -> Quaternion Normalize/1
  Quaternion Normalize/1 -> IC/1, q_i2b_#_4/1
  IC1/1 -> dynamics/2(rate)
  IC/1 -> dynamics/1(q)
  dynamics/1(d_q) -> Integrator/1
  cont_b_Nm_3/1 -> dynamics/3(t_cont)

== system lib_env/Environment&Dynamics/SRP ==
  sat2sun_i_km_3 : Inport
  sunflag_#_#_1 : Inport  Port=2
  q_i2b_#_4 : Inport  Port=3
  area_#_m^2_1 : Inport  Port=4
  Enable : EnablePort
  CR : Constant  Value=CR
  Normalize Vector : vrlib/Utilities/Normalize Vector  SystemSampleTime=-1  maxzero=0
  Quaternion Rotation2 : aerolibutil/Quaternion Rotation  SystemSampleTime=-1
  SRP : Stateflow chart  TreatAsAtomicUnit=on
  arm : Constant  Value=arm
  cross : lib_util/cross  SystemSampleTime=-1
  pSR : Constant  Value=pSR
  SRP_b_Nm_3 : Outport  InitialOutput=[0; 0; 0]
  wires:
  area_#_m^2_1/1 -> SRP/5(A)
  sunflag_#_#_1/1 -> SRP/2(flag)
  sat2sun_i_km_3/1 -> Normalize Vector/1
  q_i2b_#_4/1 -> Quaternion Rotation2/1
  cross/1 -> SRP_b_Nm_3/1
  Quaternion Rotation2/1 -> cross/2
  arm/1 -> cross/1
  SRP/1(F) -> Quaternion Rotation2/2  "[N]"
  CR/1 -> SRP/4(CR)
  pSR/1 -> SRP/3(pSR)
  Normalize Vector/1 -> SRP/1(r)

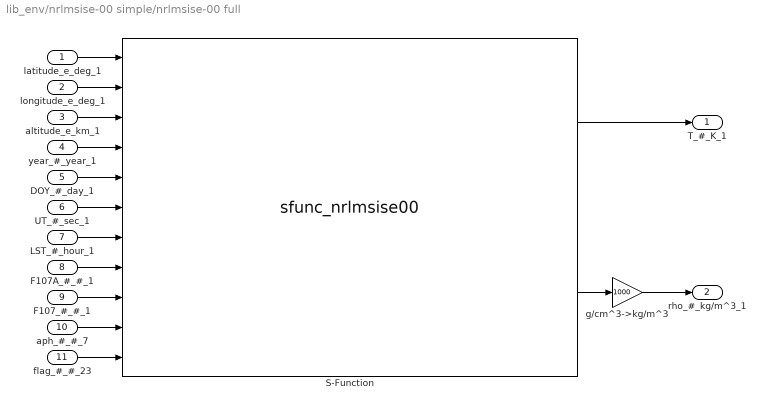
== system lib_env/nrlmsise-00 simple/nrlmsise-00 full ==
  latitude_e_deg_1 : Inport
  longitude_e_deg_1 : Inport  Port=2
  altitude_e_km_1 : Inport  Port=3
  year_#_year_1 : Inport  Port=4
  DOY_#_day_1 : Inport  Port=5
  UT_#_sec_1 : Inport  Port=6
  LST_#_hour_1 : Inport  Port=7
  F107A_#_#_1 : Inport  Port=8
  F107_#_#_1 : Inport  Port=9
  aph_#_#_7 : Inport  Port=10
  flag_#_#_23 : Inport  Port=11
  S-Function : S-Function  FunctionName=sfunc_nrlmsise00  EnableBusSupport=off
  g/cm^3->kg/m^3 : Gain  Gain=1000
  T_#_K_1 : Outport
  rho_#_kg/m^3_1 : Outport  Port=2
  wires:
  S-Function/2 -> g/cm^3->kg/m^3/1
  latitude_e_deg_1/1 -> S-Function/1
  longitude_e_deg_1/1 -> S-Function/2
  altitude_e_km_1/1 -> S-Function/3
  S-Function/1 -> T_#_K_1/1
  year_#_year_1/1 -> S-Function/4
  DOY_#_day_1/1 -> S-Function/5
  UT_#_sec_1/1 -> S-Function/6
  LST_#_hour_1/1 -> S-Function/7
  F107A_#_#_1/1 -> S-Function/8
  g/cm^3->kg/m^3/1 -> rho_#_kg/m^3_1/1
  F107_#_#_1/1 -> S-Function/9
  aph_#_#_7/1 -> S-Function/10
  flag_#_#_23/1 -> S-Function/11

== matlab function OEtoSATPOS/calc_TA_R ==
  data: ele output double; th output double; OE input double; r output double; R output double
function [ele,th,r,R] = MOE_(OE)
%#codegen
TOLERANCE=1.0e-10;

a=OE(1);         % semimajor axis [km]
e=OE(2);         % eccentricity
i=OE(3); % inclination [rad] -2*pi*floor(OE(1,4)/2/pi)
W=OE(4)-2*pi*floor(OE(4)/2/pi); % right ascension of the ascending node [rad] 
ww=OE(5)-2*pi*floor(OE(5)/2/pi); % argument of perigee [rad] 
M=OE(6)-2*pi*floor(OE(6)/2/pi); % mean anomaly at epoch [rad]
% if e < 0
%         e=-e;
%         ww=ww+pi;
%         ww=ww-2*pi*floor(ww/2/pi);
%         M=M+pi;
%         M=M-2*pi*floor(M/2/pi);
% end
ele=[a,e,i,W,ww,M];

q=a*(1-e);       % perigee distance [km]

%%%%%%%%%%%%%%%%%%%%%%%%%%%%%%%%%%%%%%%%%%%%%%%%%%%%%%%%%%%%%%%%%%%%%%%%%%%
%     calculate true anomaly th                                           %
%     calculate true distance r                                           %
%%%%%%%%%%%%%%%%%%%%%%%%%%%%%%%%%%%%%%%%%%%%%%%%%%%%%%%%%%%%%%%%%%%%%%%%%%%

if ( e == 0.0 )
    th =M;
    r=a;
elseif ( e == 1.0 )
    s = M;
      s2 = s * s;
      s3 = s2 * s;
      s = ( 2.0 * s3 + M ) / ( 3.0 * ( s2 + 1.0 ) );
      delta = s3 + 3.0 * s - M;    
    while ( abs ( delta ) > TOLERANCE )
      s2 = s * s;
      s3 = s2 * s;
      s = ( 2.0 * s3 + M ) / ( 3.0 * ( s2 + 1.0 ) );
      delta = s3 + 3.0 * s - M;
    end
    th = 2.0 * atan ( s );
    r = q * ( 1.0 + s2 );
else
    M = M-2*pi*floor(M/2/pi);
    ea = M;
    delta = ea - e * sin ( ea ) - M;    
    while ( abs ( delta ) > TOLERANCE )
      ea = ea- delta / ( 1.0 - e * cos ( ea ) );
      delta = ea - e * sin ( ea ) - M;      
    end
    th = 2.0 * atan ( sqrt ( ( 1.0 + e ) / ( 1.0 - e ) ) * tan ( ea / 2.0 ) );
    r = q * ( 1.0 + e ) / ( 1.0 + e * cos ( th ) ); 
end
  
  th=th-2*pi*floor(th/2/pi);    

% calculate DCM inertia to orbit  
  
  u = ww + th;

  cu = cos (u); ci = cos (i); cn = cos (W); 
  su = sin (u); si = sin (i); sn = sin (W); 

  R=zeros(3);
  
  R(1,1) = - su * ci * sn + cu * cn; %/* (R)_11 */
  R(2,1) = - su * ci * cn - cu * sn; %/* (R)_21 */ 
  R(3,1) =   su * si;                %/* (R)_31 */
  R(1,2) =   cu * ci * sn +su * cn;  %/* (R)_12 */
  R(2,2) =   cu * ci * cn -su * sn;  %/* (R)_22 */
  R(3,2) = - si * cu;                %/* (R)_32 */
  R(1,3) =   sn * si;                %/* (R)_13 */
  R(2,3) =   cn * si;                %/* (R)_23 */
  R(3,3) =   ci;                     %/* (R)_33 */
